simulink model "testExample_R2019b"  (R2019b)
settings: Solver=ode4  StartTime=0.0  StopTime=Inf  FixedStep=0.005  RelTol=1e-3
InitFcn:
  | [~, check_startup] = system('QPROCESS "VRNS_0.0.2.exe">NUL | IF %ERRORLEVEL% EQU 0 ECHO 666');
  | if(contains(check_startup, '.exe'))
  |     dos('C:/Program Files/VehicleRoadNoiseSimulator/VRNS_0.0.2.exe &');
  | end
StopFcn:
  | u1=udp('127.0.0.1','RemotePort',8351,'LocalPort',8341);
  | fopen(u1);
  | fprintf(u1, ['rd1sd000',226,210,205,201,199,197,196,136,136,136,226,210,205,201,199,197,196,136,136,136]);
  | fclose(u1);
libraries: etargetslib x1, instrumentlib x1
PauseFcn:
  | u1=udp('127.0.0.1','RemotePort',8351,'LocalPort',8341);
  | fopen(u1);
  | fprintf(u1, ['rd1sd000',226,210,205,201,199,197,196,136,136,136,226,210,205,201,199,197,196,136,136,136]);
  | fclose(u1);
settings Model: EnablePacing=on  Creator=TK-V  LastModifiedBy=TK-V
settings DebuggingCC: SFMachineParentedDataDiag=error

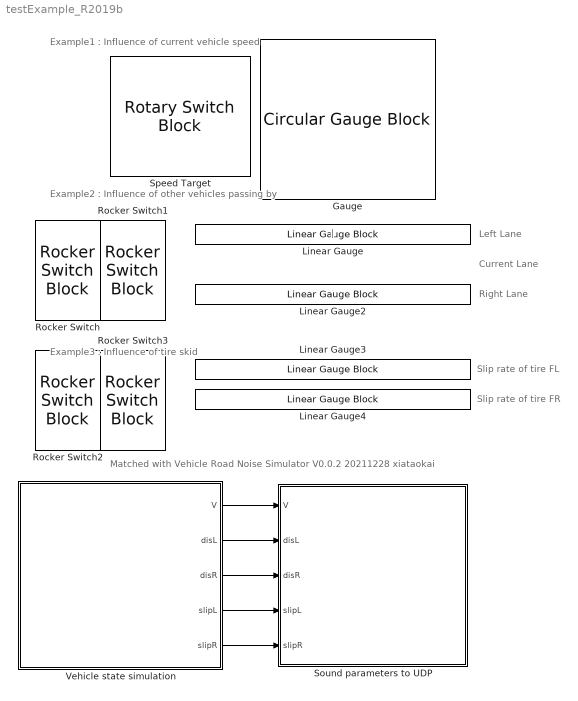
== system testExample_R2019b ==
  note: Matched with Vehicle Road Noise Simulator V0.0.2 20211228 xiataokai
  note: |
  note: Left Lane
  note: Example1：Influence of current vehicle speed
  note: Example2：Influence of other vehicles passing by
  note: Example3：Influence of tire skid
  note: Current Lane
  note: Right Lane
  note: Slip rate of tire FL
  note: Slip rate of tire FR
  Gauge : CircularGaugeBlock  LabelPosition=Bottom  ScaleMax=150  TickInterval=10
  Linear Gauge : LinearGaugeBlock  LabelPosition=Hide  ScaleMin=-100  TickInterval=20
  Linear Gauge2 : LinearGaugeBlock  LabelPosition=Hide  ScaleMin=-100  TickInterval=20
  Linear Gauge3 : LinearGaugeBlock  LabelPosition=Hide  ScaleMin=-0.5  ScaleMax=4.5  TickInterval=0.5
  Linear Gauge4 : LinearGaugeBlock  LabelPosition=Hide  ScaleMin=-0.5  ScaleMax=4.5  TickInterval=0.5
  Rocker Switch{,1..3} (4 alike) : RockerSwitchBlock  LabelPosition=Bottom
      settings: Values={{'Off', 'On'}, [0 1]}
  Sound parameters to UDP : Subsystem
  Speed Target : RotarySwitchBlock  LabelPosition=Hide
      settings: Values={{'0', '20', '40', '60', '80', '100', '120'}, [0 20 40 60 80 100 120]}
  Vehicle state simulation : Subsystem
  wires:
  Vehicle state simulation/1(V) -> Sound parameters to UDP/1(V)
  Vehicle state simulation/2(disL) -> Sound parameters to UDP/2(disL)
  Vehicle state simulation/3(disR) -> Sound parameters to UDP/3(disR)
  Vehicle state simulation/4(slipL) -> Sound parameters to UDP/4(slipL)
  Vehicle state simulation/5(slipR) -> Sound parameters to UDP/5(slipR)

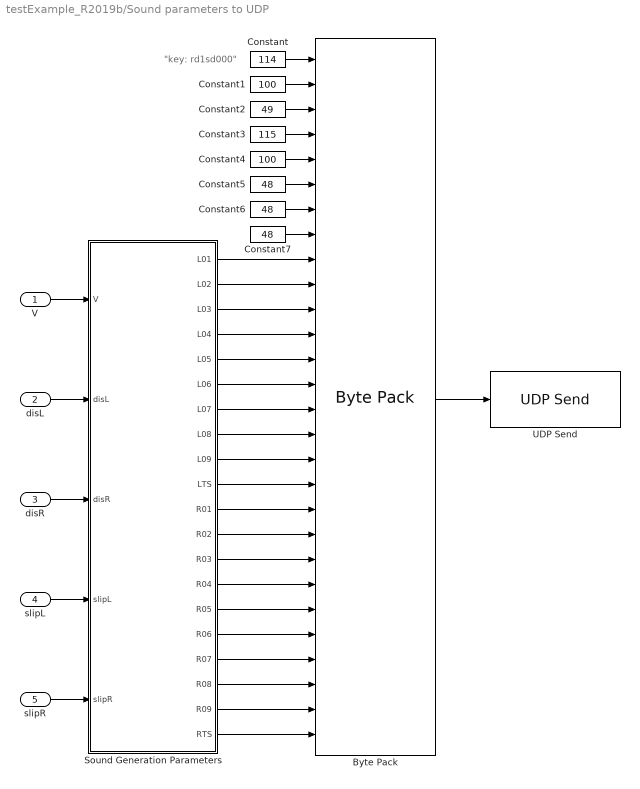
== system testExample_R2019b/Sound parameters to UDP ==
  note: "key: rd1sd000"
  V : Inport
  disL : Inport  Port=2
  disR : Inport  Port=3
  slipL : Inport  Port=4
  slipR : Inport  Port=5
  Byte Pack : etargetslib/Byte Pack  datatypes=[repmat({'uint8'},1,8),repmat({'int8'},1,20)]  byteAlign=1
  Constant : Constant  Value=114  OutDataTypeStr=uint8
  Constant1 : Constant  Value=100  OutDataTypeStr=uint8
  Constant2 : Constant  Value=49  OutDataTypeStr=uint8
  Constant3 : Constant  Value=115  OutDataTypeStr=uint8
  Constant4 : Constant  Value=100  OutDataTypeStr=uint8
  Constant5 : Constant  Value=48  OutDataTypeStr=uint8
  Constant6 : Constant  Value=48  OutDataTypeStr=uint8
  Constant7 : Constant  Value=48  OutDataTypeStr=uint8
  Sound Generation Parameters : MATLAB Function  TreatAsAtomicUnit=on
  UDP Send : instrumentlib/UDP Send  Host=127.0.0.1  Port=8351  LocalPort=-1  EnablePortSharing=off  ByteOrder=BigEndian  OutputDatagramPacketSize=28  EnableBlockingMode=on  LocalAddress=0.0.0.0
  wires:
  Constant2/1 -> Byte Pack/3
  Byte Pack/1 -> UDP Send/1
  Constant6/1 -> Byte Pack/7
  Sound Generation Parameters/18(R08) -> Byte Pack/26
  Sound Generation Parameters/11(R01) -> Byte Pack/19
  Sound Generation Parameters/9(L09) -> Byte Pack/17
  Constant7/1 -> Byte Pack/8
  Sound Generation Parameters/3(L03) -> Byte Pack/11
  Sound Generation Parameters/20(RTS) -> Byte Pack/28
  Sound Generation Parameters/2(L02) -> Byte Pack/10
  Sound Generation Parameters/10(LTS) -> Byte Pack/18
  Constant5/1 -> Byte Pack/6
  Constant3/1 -> Byte Pack/4
  Sound Generation Parameters/14(R04) -> Byte Pack/22
  Sound Generation Parameters/7(L07) -> Byte Pack/15
  Constant/1 -> Byte Pack/1
  Sound Generation Parameters/17(R07) -> Byte Pack/25
  Sound Generation Parameters/16(R06) -> Byte Pack/24
  slipR/1 -> Sound Generation Parameters/5(slipR)
  V/1 -> Sound Generation Parameters/1(V)
  Sound Generation Parameters/19(R09) -> Byte Pack/27
  Sound Generation Parameters/6(L06) -> Byte Pack/14
  Sound Generation Parameters/4(L04) -> Byte Pack/12
  Constant4/1 -> Byte Pack/5
  slipL/1 -> Sound Generation Parameters/4(slipL)
  Sound Generation Parameters/13(R03) -> Byte Pack/21
  Sound Generation Parameters/1(L01) -> Byte Pack/9
  Sound Generation Parameters/5(L05) -> Byte Pack/13
  Constant1/1 -> Byte Pack/2
  Sound Generation Parameters/15(R05) -> Byte Pack/23
  disR/1 -> Sound Generation Parameters/3(disR)
  Sound Generation Parameters/8(L08) -> Byte Pack/16
  disL/1 -> Sound Generation Parameters/2(disL)
  Sound Generation Parameters/12(R02) -> Byte Pack/20

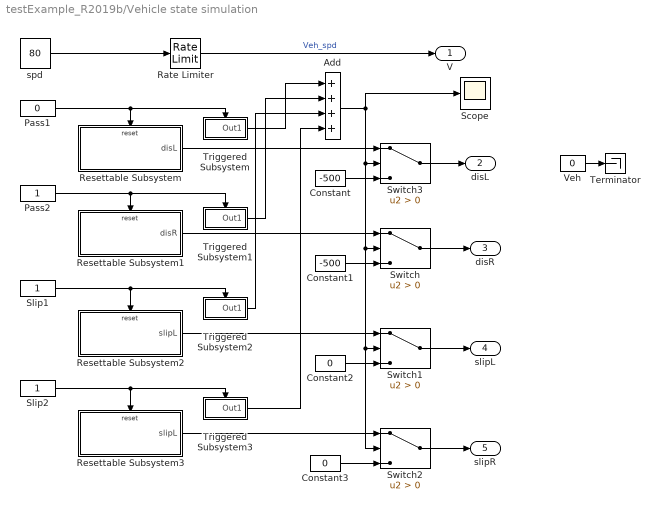
== system testExample_R2019b/Vehicle state simulation ==
  Add : Sum  Inputs=++++
  Constant : Constant  Value=-500
  Constant1 : Constant  Value=-500
  Constant2 : Constant  Value=0
  Constant3 : Constant  Value=0
  Pass1 : Constant  Value=0
  Pass2 : Constant
  Rate Limiter : RateLimiter  RisingSlewLimit=10  FallingSlewLimit=-10  SampleTimeMode=inherited
  Resettable Subsystem : Subsystem  TreatAsAtomicUnit=on
  Resettable Subsystem1 : Subsystem  TreatAsAtomicUnit=on
  Resettable Subsystem2 : Subsystem  TreatAsAtomicUnit=on
  Resettable Subsystem3 : Subsystem  TreatAsAtomicUnit=on
  Scope : Scope
  Slip1 : Constant
  Slip2 : Constant
  Switch{,1..3} (4 alike) : Switch  Criteria=u2 > Threshold
  Terminator : Terminator
  Triggered Subsystem : Subsystem  TreatAsAtomicUnit=on
  Triggered Subsystem1 : Subsystem  TreatAsAtomicUnit=on
  Triggered Subsystem2 : Subsystem  TreatAsAtomicUnit=on
  Triggered Subsystem3 : Subsystem  TreatAsAtomicUnit=on
  Veh : Constant  Value=0
  spd : Constant  Value=80
  V : Outport
  disL : Outport  Port=2
  disR : Outport  Port=3
  slipL : Outport  Port=4
  slipR : Outport  Port=5
  wires:
  Resettable Subsystem/1(disL) -> Switch3/1
  Rate Limiter/1 -> V/1  "Veh_spd"
  spd/1 -> Rate Limiter/1
  Pass1/1 -> Resettable Subsystem/Reset, Triggered Subsystem/Trigger
  Pass2/1 -> Resettable Subsystem1/Reset, Triggered Subsystem1/Trigger
  Resettable Subsystem1/1(disR) -> Switch/1
  Resettable Subsystem2/1(slipL) -> Switch1/1
  Slip1/1 -> Triggered Subsystem2/Trigger, Resettable Subsystem2/Reset
  Slip2/1 -> Triggered Subsystem3/Trigger, Resettable Subsystem3/Reset
  Resettable Subsystem3/1(slipL) -> Switch2/1
  Switch/1 -> disR/1
  Switch1/1 -> slipL/1
  Switch2/1 -> slipR/1
  Switch3/1 -> disL/1
  Constant1/1 -> Switch/3
  Constant/1 -> Switch3/3
  Constant3/1 -> Switch2/3
  Constant2/1 -> Switch1/3
  Add/1 -> Scope/1, Switch2/2, Switch1/2, Switch/2, Switch3/2
  Triggered Subsystem/1(Out1) -> Add/1
  Triggered Subsystem1/1(Out1) -> Add/2
  Triggered Subsystem2/1(Out1) -> Add/3
  Triggered Subsystem3/1(Out1) -> Add/4
  Veh/1 -> Terminator/1

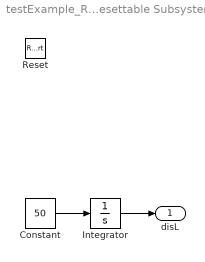
== system testExample_R2019b/Vehicle state simulation/Resettable Subsystem ==
  Reset : ResetPort  DisableCoverage=on  ResetTriggerType=either
  Constant : Constant  Value=50
  Integrator : Integrator  InitialCondition=-100  LimitOutput=on  UpperSaturationLimit=500  LowerSaturationLimit=-100
  disL : Outport
  wires:
  Integrator/1 -> disL/1
  Constant/1 -> Integrator/1

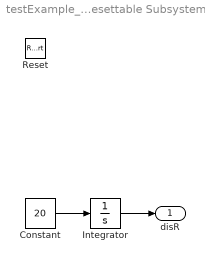
== system testExample_R2019b/Vehicle state simulation/Resettable Subsystem1 ==
  Reset : ResetPort  DisableCoverage=on  ResetTriggerType=either
  Constant : Constant  Value=20
  Integrator : Integrator  InitialCondition=-100  LimitOutput=on  UpperSaturationLimit=500  LowerSaturationLimit=-100
  disR : Outport
  wires:
  Integrator/1 -> disR/1
  Constant/1 -> Integrator/1

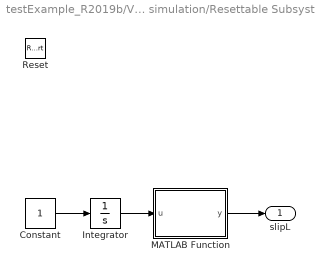
== system testExample_R2019b/Vehicle state simulation/Resettable Subsystem2 ==
  Reset : ResetPort  DisableCoverage=on  ResetTriggerType=either
  Constant : Constant
  Integrator : Integrator  UpperSaturationLimit=200  LowerSaturationLimit=-200
  MATLAB Function : MATLAB Function  TreatAsAtomicUnit=on
  slipL : Outport
  wires:
  Integrator/1 -> MATLAB Function/1(u)
  Constant/1 -> Integrator/1
  MATLAB Function/1(y) -> slipL/1

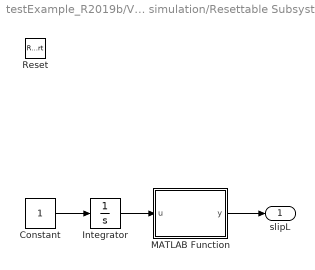
== system testExample_R2019b/Vehicle state simulation/Resettable Subsystem3 ==
  Reset : ResetPort  DisableCoverage=on  ResetTriggerType=either
  Constant : Constant
  Integrator : Integrator  UpperSaturationLimit=200  LowerSaturationLimit=-200
  MATLAB Function : MATLAB Function  TreatAsAtomicUnit=on
  slipL : Outport
  wires:
  Integrator/1 -> MATLAB Function/1(u)
  Constant/1 -> Integrator/1
  MATLAB Function/1(y) -> slipL/1

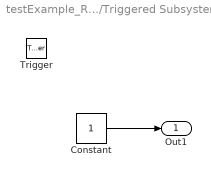
== system testExample_R2019b/Vehicle state simulation/Triggered Subsystem ==
  Trigger : TriggerPort  TriggerType=either  VariantControl=(inherit)
  Constant : Constant
  Out1 : Outport  InitialOutput=0
  wires:
  Constant/1 -> Out1/1

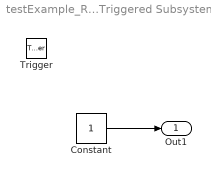
== system testExample_R2019b/Vehicle state simulation/Triggered Subsystem1 ==
  Trigger : TriggerPort  TriggerType=either  VariantControl=(inherit)
  Constant : Constant
  Out1 : Outport  InitialOutput=0
  wires:
  Constant/1 -> Out1/1

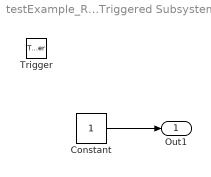
== system testExample_R2019b/Vehicle state simulation/Triggered Subsystem2 ==
  Trigger : TriggerPort  TriggerType=either  VariantControl=(inherit)
  Constant : Constant
  Out1 : Outport  InitialOutput=0
  wires:
  Constant/1 -> Out1/1

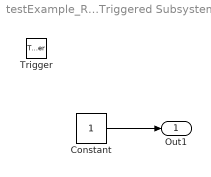
== system testExample_R2019b/Vehicle state simulation/Triggered Subsystem3 ==
  Trigger : TriggerPort  TriggerType=either  VariantControl=(inherit)
  Constant : Constant
  Out1 : Outport  InitialOutput=0
  wires:
  Constant/1 -> Out1/1

== matlab function testExample_R2019b/Vehicle state simulation/Resettable Subsystem2/MATLAB Function ==
  data: u input; y output
function y = slp(u)

V = [0, 0; 1, 0.2; 2, 1; 3, 4; 5, 1; 6, 0];

y = intMap1(V, u);

end


% 1D-Map interp
function v1 = intMap1(V, x0)
if x0 <= V(1,1)
    v1 = V(1,2);
elseif x0 >= V(end,1)
    v1 = V(end,2);
else
    for i = 1:size(V,1)-1
        if V(i+1,1) > x0; break; end
    end
    v1 = V(i,2)*(V(i+1,1)-x0)/(V(i+1,1)-V(i,1))+V(i+1,2)*(x0-V(i,1))/(V(i+1,1)-V(i,1));
end
end

== matlab function testExample_R2019b/Sound parameters to UDP/Sound Generation Parameters ==
  data: V input; L01 output; disL input; disR input; slipL input; slipR input; L02 output; L03 output; L04 output; L05 output; L06 output; L07 output; L08 output; L09 output; LTS output; R01 output; R02 output; R03 output; R04 output; R05 output; R06 output; R07 output; R08 output; R09 output; RTS output
% Vehicle Road Noise Parameter Calculation
% Matched with Vehicle Road Noise Simulator V0.0.2
% V0.0.1 20211228 xiataokai

function [L01, L02, L03, L04, L05, L06, L07, L08, L09, LTS,...
    R01, R02, R03, R04, R05, R06, R07, R08, R09, RTS] = sgp(V, disL, disR, slipL, slipR)
% Minimum sound
M = -120.0;

% Road noise caused by local vehicle speed 
V01_table = [0.0, -30.0; 40.0, -20.0; 120.0, -10.0];
V02_table = [0.0, -46.0; 30.0, -10.0; 40.0, -6.0; 120.0, -10.0];
V03_table = [0.0, -51.0; 60.0, -10.0; 120.0, -5.0];
V04_table = [0.0, -55.0; 70.0, -9.0; 120.0, -13.0];
V05_table = [0.0, -57.0; 80.0, -12.0; 120.0, -6.0];
V06_table = [0.0, -59.0; 90.0, -23.0; 120.0, -16.0];
V07_table = [0.0, -60.0; 100.0, -23.0; 120.0, -16.0];
V08_table = [0.0, -62.0; 110.0, -21.0; 120.0, -20.0];
V09_table = [0.0, -63.0; 120.0, -26.0];

% Road noise caused by vehicle passing-by
d0 = 4;
D06_fun = @(d) -0+30/log(10)*log(d0/sqrt(d.^2+d0.^2));
D07_fun = @(d) 3+30/log(10)*log(d0/sqrt(d.^2+d0.^2));
D08_fun = @(d) 3+30/log(10)*log(d0/sqrt(d.^2+d0.^2));

% Road noise caused by tire slip
S10_table = [0, -120; 0.2, -40; 0.4, -20; 0.8, -12; 1, -2];

% Noise mixing
L01 = int8(gain2db( db2gain(M) + db2gain(intMap1(V01_table, V)) ));
L02 = int8(gain2db( db2gain(M) + db2gain(intMap1(V02_table, V)) ));
L03 = int8(gain2db( db2gain(M) + db2gain(intMap1(V03_table, V)) ));
L04 = int8(gain2db( db2gain(M) + db2gain(intMap1(V04_table, V)) ));
L05 = int8(gain2db( db2gain(M) + db2gain(intMap1(V05_table, V)) ));
L06= int8(gain2db( db2gain(M) + db2gain(intMap1(V06_table, V)) + db2gain(D06_fun(disL)) ));
L07 = int8(gain2db( db2gain(M) + db2gain(intMap1(V07_table, V)) + db2gain(D07_fun(disL)) ));
L08 = int8(gain2db( db2gain(M) + db2gain(intMap1(V08_table, V)) + db2gain(D08_fun(disL)) ));
L09 = int8(gain2db( db2gain(M) + db2gain(intMap1(V09_table, V)) ));
LTS = int8(gain2db( db2gain(M) + db2gain(intMap1(S10_table, slipL))));

R01 = int8(gain2db( db2gain(M) + db2gain(intMap1(V01_table, V)) ));
R02 = int8(gain2db( db2gain(M) + db2gain(intMap1(V02_table, V)) ));
R03 = int8(gain2db( db2gain(M) + db2gain(intMap1(V03_table, V)) ));
R04 = int8(gain2db( db2gain(M) + db2gain(intMap1(V04_table, V)) ));
R05 = int8(gain2db( db2gain(M) + db2gain(intMap1(V05_table, V)) ));
R06= int8(gain2db( db2gain(M) + db2gain(intMap1(V06_table, V)) + db2gain(D06_fun(disR)) ));
R07 = int8(gain2db( db2gain(M) + db2gain(intMap1(V07_table, V)) + db2gain(D07_fun(disR)) ));
R08 = int8(gain2db( db2gain(M) + db2gain(intMap1(V08_table, V)) + db2gain(D08_fun(disR)) ));
R09 = int8(gain2db( db2gain(M) + db2gain(intMap1(V09_table, V)) ));
RTS = int8(gain2db( db2gain(M) + db2gain(intMap1(S10_table, slipR))));
end

% Gain to dB
function gain = db2gain(db)
    gain = exp(log(10)*db/20);
end

% dB to Gain
function db = gain2db(gain)
    db = min(0,max(-120, round(log(gain)/log(10)*20)));
end

% 1D-Map interp
function v1 = intMap1(V, x0)
if x0 <= V(1,1)
    v1 = V(1,2);
elseif x0 >= V(end,1)
    v1 = V(end,2);
else
    for i = 1:size(V,1)-1
        if V(i+1,1) > x0; break; end
    end
    v1 = V(i,2)*(V(i+1,1)-x0)/(V(i+1,1)-V(i,1))+V(i+1,2)*(x0-V(i,1))/(V(i+1,1)-V(i,1));
end
end

== matlab function testExample_R2019b/Vehicle state simulation/Resettable Subsystem3/MATLAB Function ==
  data: u input; y output
function y = slp(u)

V = [0, 0; 1, 0.2; 2, 1; 3, 4; 5, 1; 6, 0];

y = intMap1(V, u);

end


% 1D-Map interp
function v1 = intMap1(V, x0)
if x0 <= V(1,1)
    v1 = V(1,2);
elseif x0 >= V(end,1)
    v1 = V(end,2);
else
    for i = 1:size(V,1)-1
        if V(i+1,1) > x0; break; end
    end
    v1 = V(i,2)*(V(i+1,1)-x0)/(V(i+1,1)-V(i,1))+V(i+1,2)*(x0-V(i,1))/(V(i+1,1)-V(i,1));
end
end
